simulink model "softMBD"  (R2025b)
settings: Solver=FixedStepAuto  StartTime=0.0  StopTime=30  FixedStep=0.005  RelTol=1e-3
values from neighbouring files (symbols this model uses):
  FPV_mass = 0.8    [Soft.m]
  g = 9.81    [Soft.m]
  ks = 0    [Soft.m]
  p_0 = 1013.25    [Soft.m]
  Q2Ts = forcetomotors()    [Soft.m]    (also in forcetomotors.m = inv(Ts2Q))
  takeOffDuration = 2    [Soft.m]
  Ts = 0.005    [Soft.m]
undefined symbols (not defined in the file or in its folder): CdA, DiscIntNeverNeededParam, kd_pq, kd_pr, kd_y, ki_pq, ki_pr, ki_y, kp_pq, kp_pr, kp_y, pInitialization, rho
libraries: simulink x37, discretizing x11, slpidlib x2, SignalEditorBlockLib x1, simulink_extras x1, shared6dof x1, dynamicsLibrary x1, aerolibasang x1, aerolibnav x1
(part 10 of 20)

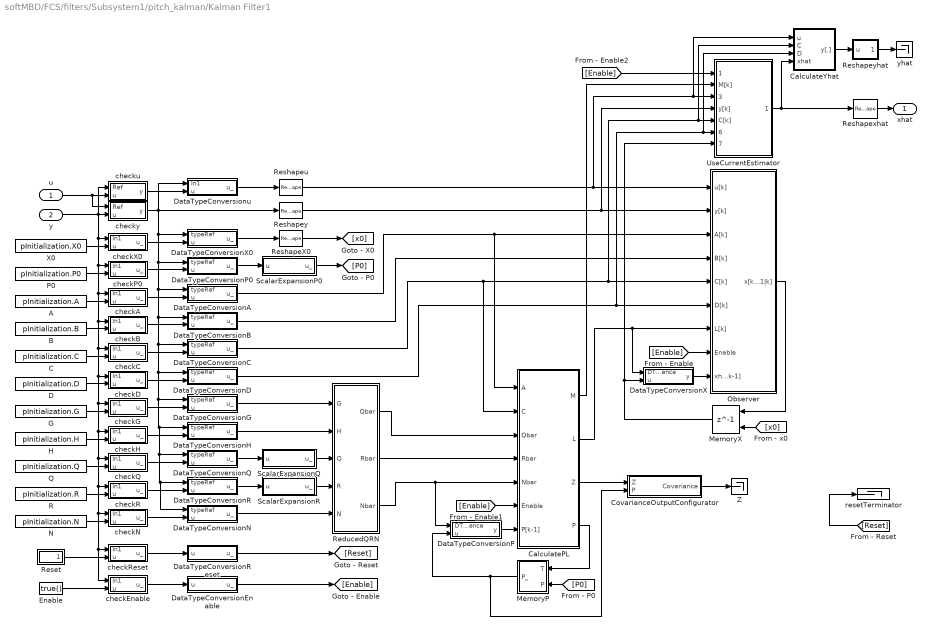
== system softMBD/FCS/filters/Subsystem1/pitch_kalman/Kalman Filter1 ==
  u : Inport
  y : Inport  Port=2
  A : Constant  Value=pInitialization.A  VectorParams1D=off  OutDataTypeStr=Inherit: Inherit via back propagation
  B : Constant  Value=pInitialization.B  VectorParams1D=off  OutDataTypeStr=Inherit: Inherit via back propagation
  C : Constant  Value=pInitialization.C  VectorParams1D=off  OutDataTypeStr=Inherit: Inherit via back propagation
  CalculatePL : Subsystem  AncestorBlock=ctrlSharedLib/KalmanFilterUtilities/ConstantPL  mask(ctrlKalmanFilterConstantPL){}
  CalculateYhat : Subsystem  AncestorBlock=ctrlSharedLib/KalmanFilterUtilities/DontCalculateYhat  mask(ctrlKalmanFilterDontCalculateYhat){}
  CovarianceOutputConfigurator : Subsystem
  D : Constant  Value=pInitialization.D  VectorParams1D=off  OutDataTypeStr=Inherit: Inherit via back propagation
  DataTypeConversionA : Subsystem  AncestorBlock=ctrlSharedLib/Utilities/DataTypeDuplicateAndOutput  mask(ctrlDataTypeDuplicateAndOutput){}
  DataTypeConversionB : Subsystem  AncestorBlock=ctrlSharedLib/Utilities/DataTypeDuplicateAndOutput  mask(ctrlDataTypeDuplicateAndOutput){}
  DataTypeConversionC : Subsystem  AncestorBlock=ctrlSharedLib/Utilities/DataTypeDuplicateAndOutput  mask(ctrlDataTypeDuplicateAndOutput){}
  DataTypeConversionD : Subsystem  AncestorBlock=ctrlSharedLib/Utilities/DataTypeDuplicateAndOutput  mask(ctrlDataTypeDuplicateAndOutput){}
  DataTypeConversionEnable : Subsystem  AncestorBlock=ctrlSharedLib/Utilities/PassInputThrough
  DataTypeConversionG : Subsystem  AncestorBlock=ctrlSharedLib/Utilities/DataTypeDuplicateAndOutput  mask(ctrlDataTypeDuplicateAndOutput){}
  DataTypeConversionH : Subsystem  AncestorBlock=ctrlSharedLib/Utilities/DataTypeDuplicateAndOutput  mask(ctrlDataTypeDuplicateAndOutput){}
  DataTypeConversionN : Subsystem  AncestorBlock=ctrlSharedLib/Utilities/DataTypeDuplicateAndOutput  mask(ctrlDataTypeDuplicateAndOutput){}
  DataTypeConversionP : Subsystem  AncestorBlock=|  mask(Conversion Inherited){ConvertRealWorld=Real World Value, RndMeth=Floor, DoSatur=off}
      | simulink/Signal
      | Attributes/Data Type
      | Conversion
      | Inherited
      mask prompts: ConvertRealWorld "Simulink:masks:InputAndOutputToHaveEqual_MP"; RndMeth "Simulink:masks:IntegerRoundingMode_MP"; DoSatur "Simulink:masks:SaturateToMaxOrMinWhenOverflowsOccur_MP"
      mask help: Simulink:masks:ConversionInherited_MD
      mask init:
      | rndMethCell = {'Ceiling','Convergent','Floor','Nearest','Round','Simplest','Zero'};
      | onOffCell = {'off','on'};
      | RWVvsSICell = { 'Real World Value','Stored Integer'};
      | set_param([gcb,'/Conversion'],'RndMeth',rndMethCell{RndMeth},...
      |                                 'DoSatur',onOffCell{DoSatur+1},...
      |                                 'ConvertRealWorld',RWVvsSICell{ConvertRealWorld});
      mask TypeOptions ConvertRealWorld: Simulink:masks:RealWorldValue | Simulink:masks:StoredInteger
      mask TypeOptions RndMeth: Simulink:masks:Ceiling | Simulink:masks:Convergent | Simulink:masks:Floor | Simulink:masks:Nearest | Simulink:masks:Round | Simulink:masks:Simplest | Simulink:masks:Zero
      mask Display:
      | port_label('Input',2,'u');
      | port_label('Output',1,'y');
      |     if(get_param(gcbh,'ConvertRealWorld') == "Stored Integer")
      |        disp('SI')
      |     else
      |        disp('Convert')
      |     end
  DataTypeConversionP0 : Subsystem  AncestorBlock=ctrlSharedLib/Utilities/DataTypeDuplicateAndOutput  mask(ctrlDataTypeDuplicateAndOutput){}
  DataTypeConversionQ : Subsystem  AncestorBlock=ctrlSharedLib/Utilities/DataTypeDuplicateAndOutput  mask(ctrlDataTypeDuplicateAndOutput){}
  DataTypeConversionR : Subsystem  AncestorBlock=ctrlSharedLib/Utilities/DataTypeDuplicateAndOutput  mask(ctrlDataTypeDuplicateAndOutput){}
  DataTypeConversionReset : Subsystem  AncestorBlock=ctrlSharedLib/Utilities/PassInputThrough
  DataTypeConversionX : Subsystem  AncestorBlock=|  mask(Conversion Inherited){ConvertRealWorld=Real World Value, RndMeth=Floor, DoSatur=off}
      | simulink/Signal
      | Attributes/Data Type
      | Conversion
      | Inherited
      mask prompts: ConvertRealWorld "Simulink:masks:InputAndOutputToHaveEqual_MP"; RndMeth "Simulink:masks:IntegerRoundingMode_MP"; DoSatur "Simulink:masks:SaturateToMaxOrMinWhenOverflowsOccur_MP"
      mask help: Simulink:masks:ConversionInherited_MD
      mask init: same as softMBD/FCS/filters/Subsystem1/pitch_kalman/Kalman Filter1/DataTypeConversionP
      mask TypeOptions ConvertRealWorld: Simulink:masks:RealWorldValue | Simulink:masks:StoredInteger
      mask TypeOptions RndMeth: Simulink:masks:Ceiling | Simulink:masks:Convergent | Simulink:masks:Floor | Simulink:masks:Nearest | Simulink:masks:Round | Simulink:masks:Simplest | Simulink:masks:Zero
      mask Display:
      | port_label('Input',2,'u');
      | port_label('Output',1,'y');
      |     if(get_param(gcbh,'ConvertRealWorld') == "Stored Integer")
      |        disp('SI')
      |     else
      |        disp('Convert')
      |     end
  DataTypeConversionX0 : Subsystem  AncestorBlock=ctrlSharedLib/Utilities/DataTypeDuplicateAndOutput  mask(ctrlDataTypeDuplicateAndOutput){}
  DataTypeConversionu : Subsystem  AncestorBlock=ctrlSharedLib/KalmanFilterUtilities/PassSecondInputThrough  mask(ctrlKalmanFilterPassSecondInputThrough){}
      mask Display:
      | port_label('Input',2,'u');
      | port_label('Output',1,'y');
  Enable : Constant  Value=true()  OutDataTypeStr=boolean
  G : Constant  Value=pInitialization.G  VectorParams1D=off  OutDataTypeStr=Inherit: Inherit via back propagation
  H : Constant  Value=pInitialization.H  VectorParams1D=off  OutDataTypeStr=Inherit: Inherit via back propagation
  MemoryP : Subsystem  AncestorBlock=ctrlSharedLib/KalmanFilterUtilities/MemoryP  mask(ctrlKalmanFilterNoMemoryP){}
      mask Display:
      | port_label('Input',2,'P');
      | port_label('Output',1,'P');
  MemoryX : Delay  DelayLength=1  InitialConditionSource=Input port  SampleTime=pInitialization.Ts
      settings: InputPortMap=u0,p4
  N : Constant  Value=pInitialization.N  VectorParams1D=off  OutDataTypeStr=Inherit: Inherit via back propagation
  Observer : Subsystem
  P0 : Constant  Value=pInitialization.P0  OutDataTypeStr=Inherit: Inherit via back propagation
  Q : Constant  Value=pInitialization.Q  VectorParams1D=off  OutDataTypeStr=Inherit: Inherit via back propagation
  R : Constant  Value=pInitialization.R  VectorParams1D=off  OutDataTypeStr=Inherit: Inherit via back propagation
  ReducedQRN : Subsystem  AncestorBlock=ctrlSharedLib/KalmanFilterUtilities/NoReducedQRN  mask(ctrlKalmanFilterNoReducedQRN){}
  Reset : Subsystem  AncestorBlock=ctrlSharedLib/Utilities/Ground  mask(ctrlSharedLibGround){OutDataTypeStr=boolean, Dimensions=1}
      mask prompts: OutDataTypeStr "Simulink:blkprm_prompts:UNIFIEDDATATYPE"; Dimensions "Simulink:blkprm_prompts:SigSpecDims"
      mask TypeOptions OutDataTypeStr: Signal Specification/OutDataTypeStr
      mask TypeOptions Dimensions: Signal Specification/Dimensions
      mask DialogControl OutDataTypeStr Prompt: Data type:
      mask DialogControl Dimensions Prompt: Dimensions (-1 for inherited):
  ReshapeX0 : Reshape
  Reshapeu : Reshape
  Reshapexhat : Reshape
  Reshapey : Reshape
  Reshapeyhat : Subsystem  AncestorBlock=ctrlSharedLib/Utilities/PassInputThrough
  ScalarExpansionP0 : Subsystem  AncestorBlock=ctrlSharedLib/Utilities/PassInputThrough
  ScalarExpansionQ : Subsystem  AncestorBlock=ctrlSharedLib/Utilities/PassInputThrough
  ScalarExpansionR : Subsystem  AncestorBlock=ctrlSharedLib/Utilities/PassInputThrough
  UseCurrentEstimator : Subsystem  AncestorBlock=ctrlSharedLib/KalmanFilterUtilities/UseCurrentEstimatorZeroD  mask(ctrlKalmanFilterUseCurrentEstimatorZeroD){}
  X0 : Constant  Value=pInitialization.X0  VectorParams1D=off  OutDataTypeStr=Inherit: Inherit via back propagation
  Z : Terminator
  checkA : Subsystem  AncestorBlock=ctrlSharedLib/KalmanFilterUtilities/PassSecondInputThrough  mask(ctrlKalmanFilterPassSecondInputThrough){}
      mask Display:
      | port_label('Input',2,'u');
      | port_label('Output',1,'y');
  checkB : Subsystem  AncestorBlock=ctrlSharedLib/KalmanFilterUtilities/PassSecondInputThrough  mask(ctrlKalmanFilterPassSecondInputThrough){}
      mask Display:
      | port_label('Input',2,'u');
      | port_label('Output',1,'y');
  checkC : Subsystem  AncestorBlock=ctrlSharedLib/KalmanFilterUtilities/PassSecondInputThrough  mask(ctrlKalmanFilterPassSecondInputThrough){}
      mask Display:
      | port_label('Input',2,'u');
      | port_label('Output',1,'y');
  checkD : Subsystem  AncestorBlock=ctrlSharedLib/KalmanFilterUtilities/PassSecondInputThrough  mask(ctrlKalmanFilterPassSecondInputThrough){}
      mask Display:
      | port_label('Input',2,'u');
      | port_label('Output',1,'y');
  checkEnable : Subsystem  AncestorBlock=ctrlSharedLib/KalmanFilterUtilities/PassSecondInputThrough  mask(ctrlKalmanFilterPassSecondInputThrough){}
      mask Display:
      | port_label('Input',2,'u');
      | port_label('Output',1,'y');
  checkG : Subsystem  AncestorBlock=ctrlSharedLib/KalmanFilterUtilities/PassSecondInputThrough  mask(ctrlKalmanFilterPassSecondInputThrough){}
      mask Display:
      | port_label('Input',2,'u');
      | port_label('Output',1,'y');
  checkH : Subsystem  AncestorBlock=ctrlSharedLib/KalmanFilterUtilities/PassSecondInputThrough  mask(ctrlKalmanFilterPassSecondInputThrough){}
      mask Display:
      | port_label('Input',2,'u');
      | port_label('Output',1,'y');
  checkN : Subsystem  AncestorBlock=ctrlSharedLib/KalmanFilterUtilities/PassSecondInputThrough  mask(ctrlKalmanFilterPassSecondInputThrough){}
      mask Display:
      | port_label('Input',2,'u');
      | port_label('Output',1,'y');
  checkP0 : Subsystem  AncestorBlock=ctrlSharedLib/KalmanFilterUtilities/PassSecondInputThrough  mask(ctrlKalmanFilterPassSecondInputThrough){}
      mask Display:
      | port_label('Input',2,'u');
      | port_label('Output',1,'y');
  checkQ : Subsystem  AncestorBlock=ctrlSharedLib/KalmanFilterUtilities/PassSecondInputThrough  mask(ctrlKalmanFilterPassSecondInputThrough){}
      mask Display:
      | port_label('Input',2,'u');
      | port_label('Output',1,'y');
  checkR : Subsystem  AncestorBlock=ctrlSharedLib/KalmanFilterUtilities/PassSecondInputThrough  mask(ctrlKalmanFilterPassSecondInputThrough){}
      mask Display:
      | port_label('Input',2,'u');
      | port_label('Output',1,'y');
  checkReset : Subsystem  AncestorBlock=ctrlSharedLib/KalmanFilterUtilities/PassSecondInputThrough  mask(ctrlKalmanFilterPassSecondInputThrough){}
      mask Display:
      | port_label('Input',2,'u');
      | port_label('Output',1,'y');
  checkX0 : Subsystem  AncestorBlock=ctrlSharedLib/KalmanFilterUtilities/PassSecondInputThrough  mask(ctrlKalmanFilterPassSecondInputThrough){}
      mask Display:
      | port_label('Input',2,'u');
      | port_label('Output',1,'y');
  checku : Subsystem  AncestorBlock=ctrlSharedLib/KalmanFilterUtilities/checkSignals  mask(ctrlKalmanFilterCheckSignals){Ts=pInitialization.Ts, Ns=pInitialization.Ns, Nu=pInitialization.Nu, Nw=pInitialization.Nw, Ny=pInitialization.Ny}
      mask prompts: Ts "Sample time:"; Ns "Number of states:"; Nu "Number of inputs:"; Nw "Number of process noise inputs:"; Ny "Number of outputs:"
      mask init:
      | Ns = int32(Ns);
      | Nu = int32(Nu);
      | Nw = int32(Nw);
      | Ny = int32(Ny);
      | 
      | lineH = get_param(gcbh,'LineHandles');
      | portName = get_param(get_param(lineH.Inport(2),'SrcBlockHandle'),'Name');
      | parentBlockPath = get_param(gcbh(),'Parent');
      | parentH = get_param(parentBlockPath,'Handle');
      | isContinuousTime = strcmp(get_param(parentH,'TimeDomain'),...
      |     slsvInternal('slsvGetEnStringFromCatalog','Controllib:blocks:maskPromptKFTimeDomainCT'));
      | clear lineH;
      mask DialogControl ParametersContainer Prompt: Parameters
  checky : Subsystem  AncestorBlock=ctrlSharedLib/KalmanFilterUtilities/checkSignals  mask(ctrlKalmanFilterCheckSignals){Ts=pInitialization.Ts, Ns=pInitialization.Ns, Nu=pInitialization.Nu, Nw=pInitialization.Nw, Ny=pInitialization.Ny}
      mask prompts: Ts "Sample time:"; Ns "Number of states:"; Nu "Number of inputs:"; Nw "Number of process noise inputs:"; Ny "Number of outputs:"
      mask init: same as softMBD/FCS/filters/Subsystem1/pitch_kalman/Kalman Filter1/checku
      mask DialogControl ParametersContainer Prompt: Parameters
  resetTerminator : Terminator
  yhat : Terminator
  xhat : Outport  VectorParamsAs1DForOutWhenUnconnected=off
  wires:
  [Reset] -> resetTerminator/1
  CalculatePL/3(Z) -> CovarianceOutputConfigurator/1(Z)
  Reshapexhat/1 -> xhat/1
  Reshapeyhat/1(u_) -> yhat/1
  UseCurrentEstimator/1(xhat[k|k]) -> Reshapexhat/1, CalculateYhat/4(xhat)
  checku/1(y) -> DataTypeConversionu/2(u)
  DataTypeConversionu/1(u_) -> Reshapeu/1
  CovarianceOutputConfigurator/1(Covariance) -> Z/1
  DataTypeConversionC/1(u_) -> Observer/5(C[k]), UseCurrentEstimator/5(C[k]), CalculateYhat/2(C), CalculatePL/2(C)
  ScalarExpansionR/1(u_) -> ReducedQRN/4(R)
  ScalarExpansionQ/1(u_) -> ReducedQRN/3(Q)
  ScalarExpansionP0/1(u_) -> [P0]
  CalculatePL/4(P) -> MemoryP/1(T)
  DataTypeConversionReset/1(u_) -> [Reset]
  checkReset/1(u_) -> DataTypeConversionReset/1(u)
  checky/1(y) -> DataTypeConversionX0/1(typeRef), DataTypeConversionP0/1(typeRef), DataTypeConversionC/1(typeRef), DataTypeConversionD/1(typeRef), DataTypeConversionG/1(typeRef), DataTypeConversionH/1(typeRef), DataTypeConversionQ/1(typeRef), DataTypeConversionR/1(typeRef), DataTypeConversionN/1(typeRef), DataTypeConversionB/1(typeRef), DataTypeConversionA/1(typeRef), Reshapey/1, DataTypeConversionu/1(In1)
  ReshapeX0/1 -> [x0]
  MemoryP/1(P_) -> DataTypeConversionP/2(u), CovarianceOutputConfigurator/2(P)
  [P0] -> MemoryP/2(P)
  CalculateYhat/1(y[.]) -> Reshapeyhat/1(u)
  [Enable] -> UseCurrentEstimator/1(Enable[k])
  CalculatePL/1(M) -> UseCurrentEstimator/2(M[k])
  CalculatePL/2(L) -> Observer/7(L[k]), DataTypeConversionX/1(DTS reference)
  Reshapey/1 -> Observer/2(y[k]), UseCurrentEstimator/4(y[k])
  Reshapeu/1 -> Observer/1(u[k]), UseCurrentEstimator/3(u (unused)), CalculateYhat/1(u)
  y/1 -> checky/2(u), checku/1(Ref), checkX0/1(In1), checkP0/1(In1), checkA/1(In1), checkB/1(In1), checkC/1(In1), checkD/1(In1), checkG/1(In1), checkH/1(In1), checkQ/1(In1), checkR/1(In1), checkN/1(In1), checkReset/1(In1), checkEnable/1(In1)
  u/1 -> checku/2(u), checky/1(Ref)
  DataTypeConversionP/1(y) -> CalculatePL/7(P[k-1])
  [Enable] -> Observer/8(Enable)
  DataTypeConversionX/1(y) -> Observer/9(xhat[k|k-1])
  DataTypeConversionX0/1(u_) -> ReshapeX0/1
  [x0] -> MemoryX/2
  X0/1 -> checkX0/2(u)
  DataTypeConversionD/1(u_) -> Observer/6(D[k]), UseCurrentEstimator/6(D (unused)), CalculateYhat/3(D)
  DataTypeConversionB/1(u_) -> Observer/4(B[k])
  DataTypeConversionA/1(u_) -> Observer/3(A[k]), CalculatePL/1(A)
  checkB/1(u_) -> DataTypeConversionB/2(u)
  B/1 -> checkB/2(u)
  ReducedQRN/3(Nbar) -> CalculatePL/5(Nbar), DataTypeConversionP/1(DTS reference)
  ReducedQRN/2(Rbar) -> CalculatePL/4(Rbar)
  ReducedQRN/1(Qbar) -> CalculatePL/3(Qbar)
  checkA/1(u_) -> DataTypeConversionA/2(u)
  A/1 -> checkA/2(u)
  [Enable] -> CalculatePL/6(Enable)
  Observer/1(x[k+1|k]) -> MemoryX/1
  DataTypeConversionEnable/1(u_) -> [Enable]
  checkEnable/1(u_) -> DataTypeConversionEnable/1(u)
  Enable/1 -> checkEnable/2(u)
  DataTypeConversionP0/1(u_) -> ScalarExpansionP0/1(u)
  Reset/1(Out) -> checkReset/2(u)
  DataTypeConversionN/1(u_) -> ReducedQRN/5(N)
  checkN/1(u_) -> DataTypeConversionN/2(u)
  checkR/1(u_) -> DataTypeConversionR/2(u)
  DataTypeConversionR/1(u_) -> ScalarExpansionR/1(u)
  checkQ/1(u_) -> DataTypeConversionQ/2(u)
  DataTypeConversionQ/1(u_) -> ScalarExpansionQ/1(u)
  DataTypeConversionH/1(u_) -> ReducedQRN/2(H)
  checkH/1(u_) -> DataTypeConversionH/2(u)
  DataTypeConversionG/1(u_) -> ReducedQRN/1(G)
  checkG/1(u_) -> DataTypeConversionG/2(u)
  checkD/1(u_) -> DataTypeConversionD/2(u)
  checkC/1(u_) -> DataTypeConversionC/2(u)
  checkP0/1(u_) -> DataTypeConversionP0/2(u)
  checkX0/1(u_) -> DataTypeConversionX0/2(u)
  MemoryX/1 -> DataTypeConversionX/2(u), UseCurrentEstimator/7(xhat[k|k-1])
  N/1 -> checkN/2(u)
  R/1 -> checkR/2(u)
  Q/1 -> checkQ/2(u)
  H/1 -> checkH/2(u)
  G/1 -> checkG/2(u)
  D/1 -> checkD/2(u)
  P0/1 -> checkP0/2(u)
  C/1 -> checkC/2(u)

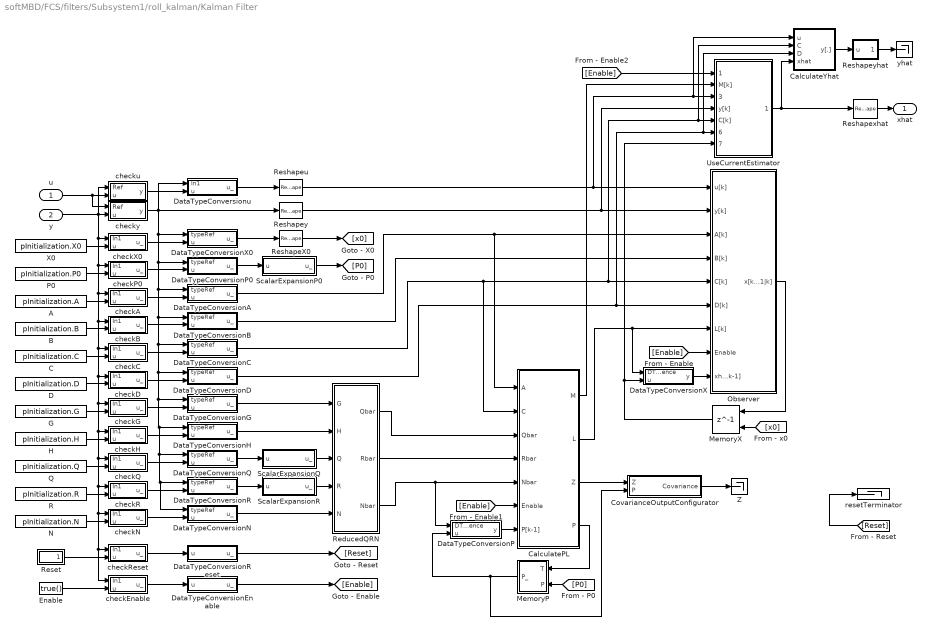
== system softMBD/FCS/filters/Subsystem1/roll_kalman/Kalman Filter ==
  u : Inport
  y : Inport  Port=2
  A : Constant  Value=pInitialization.A  VectorParams1D=off  OutDataTypeStr=Inherit: Inherit via back propagation
  B : Constant  Value=pInitialization.B  VectorParams1D=off  OutDataTypeStr=Inherit: Inherit via back propagation
  C : Constant  Value=pInitialization.C  VectorParams1D=off  OutDataTypeStr=Inherit: Inherit via back propagation
  CalculatePL : Subsystem  AncestorBlock=ctrlSharedLib/KalmanFilterUtilities/ConstantPL  mask(ctrlKalmanFilterConstantPL){}
  CalculateYhat : Subsystem  AncestorBlock=ctrlSharedLib/KalmanFilterUtilities/DontCalculateYhat  mask(ctrlKalmanFilterDontCalculateYhat){}
  CovarianceOutputConfigurator : Subsystem
  D : Constant  Value=pInitialization.D  VectorParams1D=off  OutDataTypeStr=Inherit: Inherit via back propagation
  DataTypeConversionA : Subsystem  AncestorBlock=ctrlSharedLib/Utilities/DataTypeDuplicateAndOutput  mask(ctrlDataTypeDuplicateAndOutput){}
  DataTypeConversionB : Subsystem  AncestorBlock=ctrlSharedLib/Utilities/DataTypeDuplicateAndOutput  mask(ctrlDataTypeDuplicateAndOutput){}
  DataTypeConversionC : Subsystem  AncestorBlock=ctrlSharedLib/Utilities/DataTypeDuplicateAndOutput  mask(ctrlDataTypeDuplicateAndOutput){}
  DataTypeConversionD : Subsystem  AncestorBlock=ctrlSharedLib/Utilities/DataTypeDuplicateAndOutput  mask(ctrlDataTypeDuplicateAndOutput){}
  DataTypeConversionEnable : Subsystem  AncestorBlock=ctrlSharedLib/Utilities/PassInputThrough
  DataTypeConversionG : Subsystem  AncestorBlock=ctrlSharedLib/Utilities/DataTypeDuplicateAndOutput  mask(ctrlDataTypeDuplicateAndOutput){}
  DataTypeConversionH : Subsystem  AncestorBlock=ctrlSharedLib/Utilities/DataTypeDuplicateAndOutput  mask(ctrlDataTypeDuplicateAndOutput){}
  DataTypeConversionN : Subsystem  AncestorBlock=ctrlSharedLib/Utilities/DataTypeDuplicateAndOutput  mask(ctrlDataTypeDuplicateAndOutput){}
  DataTypeConversionP : Subsystem  AncestorBlock=|  mask(Conversion Inherited){ConvertRealWorld=Real World Value, RndMeth=Floor, DoSatur=off}
      | simulink/Signal
      | Attributes/Data Type
      | Conversion
      | Inherited
      mask prompts: ConvertRealWorld "Simulink:masks:InputAndOutputToHaveEqual_MP"; RndMeth "Simulink:masks:IntegerRoundingMode_MP"; DoSatur "Simulink:masks:SaturateToMaxOrMinWhenOverflowsOccur_MP"
      mask help: Simulink:masks:ConversionInherited_MD
      mask init: same as softMBD/FCS/filters/Subsystem1/pitch_kalman/Kalman Filter1/DataTypeConversionP
      mask TypeOptions ConvertRealWorld: Simulink:masks:RealWorldValue | Simulink:masks:StoredInteger
      mask TypeOptions RndMeth: Simulink:masks:Ceiling | Simulink:masks:Convergent | Simulink:masks:Floor | Simulink:masks:Nearest | Simulink:masks:Round | Simulink:masks:Simplest | Simulink:masks:Zero
      mask Display:
      | port_label('Input',2,'u');
      | port_label('Output',1,'y');
      |     if(get_param(gcbh,'ConvertRealWorld') == "Stored Integer")
      |        disp('SI')
      |     else
      |        disp('Convert')
      |     end
  DataTypeConversionP0 : Subsystem  AncestorBlock=ctrlSharedLib/Utilities/DataTypeDuplicateAndOutput  mask(ctrlDataTypeDuplicateAndOutput){}
  DataTypeConversionQ : Subsystem  AncestorBlock=ctrlSharedLib/Utilities/DataTypeDuplicateAndOutput  mask(ctrlDataTypeDuplicateAndOutput){}
  DataTypeConversionR : Subsystem  AncestorBlock=ctrlSharedLib/Utilities/DataTypeDuplicateAndOutput  mask(ctrlDataTypeDuplicateAndOutput){}
  DataTypeConversionReset : Subsystem  AncestorBlock=ctrlSharedLib/Utilities/PassInputThrough
  DataTypeConversionX : Subsystem  AncestorBlock=|  mask(Conversion Inherited){ConvertRealWorld=Real World Value, RndMeth=Floor, DoSatur=off}
      | simulink/Signal
      | Attributes/Data Type
      | Conversion
      | Inherited
      mask prompts: ConvertRealWorld "Simulink:masks:InputAndOutputToHaveEqual_MP"; RndMeth "Simulink:masks:IntegerRoundingMode_MP"; DoSatur "Simulink:masks:SaturateToMaxOrMinWhenOverflowsOccur_MP"
      mask help: Simulink:masks:ConversionInherited_MD
      mask init: same as softMBD/FCS/filters/Subsystem1/pitch_kalman/Kalman Filter1/DataTypeConversionP
      mask TypeOptions ConvertRealWorld: Simulink:masks:RealWorldValue | Simulink:masks:StoredInteger
      mask TypeOptions RndMeth: Simulink:masks:Ceiling | Simulink:masks:Convergent | Simulink:masks:Floor | Simulink:masks:Nearest | Simulink:masks:Round | Simulink:masks:Simplest | Simulink:masks:Zero
      mask Display:
      | port_label('Input',2,'u');
      | port_label('Output',1,'y');
      |     if(get_param(gcbh,'ConvertRealWorld') == "Stored Integer")
      |        disp('SI')
      |     else
      |        disp('Convert')
      |     end
  DataTypeConversionX0 : Subsystem  AncestorBlock=ctrlSharedLib/Utilities/DataTypeDuplicateAndOutput  mask(ctrlDataTypeDuplicateAndOutput){}
  DataTypeConversionu : Subsystem  AncestorBlock=ctrlSharedLib/KalmanFilterUtilities/PassSecondInputThrough  mask(ctrlKalmanFilterPassSecondInputThrough){}
      mask Display:
      | port_label('Input',2,'u');
      | port_label('Output',1,'y');
  Enable : Constant  Value=true()  OutDataTypeStr=boolean
  G : Constant  Value=pInitialization.G  VectorParams1D=off  OutDataTypeStr=Inherit: Inherit via back propagation
  H : Constant  Value=pInitialization.H  VectorParams1D=off  OutDataTypeStr=Inherit: Inherit via back propagation
  MemoryP : Subsystem  AncestorBlock=ctrlSharedLib/KalmanFilterUtilities/MemoryP  mask(ctrlKalmanFilterNoMemoryP){}
      mask Display:
      | port_label('Input',2,'P');
      | port_label('Output',1,'P');
  MemoryX : Delay  DelayLength=1  InitialConditionSource=Input port  SampleTime=pInitialization.Ts
      settings: InputPortMap=u0,p4
  N : Constant  Value=pInitialization.N  VectorParams1D=off  OutDataTypeStr=Inherit: Inherit via back propagation
  Observer : Subsystem
  P0 : Constant  Value=pInitialization.P0  OutDataTypeStr=Inherit: Inherit via back propagation
  Q : Constant  Value=pInitialization.Q  VectorParams1D=off  OutDataTypeStr=Inherit: Inherit via back propagation
  R : Constant  Value=pInitialization.R  VectorParams1D=off  OutDataTypeStr=Inherit: Inherit via back propagation
  ReducedQRN : Subsystem  AncestorBlock=ctrlSharedLib/KalmanFilterUtilities/NoReducedQRN  mask(ctrlKalmanFilterNoReducedQRN){}
  Reset : Subsystem  AncestorBlock=ctrlSharedLib/Utilities/Ground  mask(ctrlSharedLibGround){OutDataTypeStr=boolean, Dimensions=1}
      mask prompts: OutDataTypeStr "Simulink:blkprm_prompts:UNIFIEDDATATYPE"; Dimensions "Simulink:blkprm_prompts:SigSpecDims"
      mask TypeOptions OutDataTypeStr: Signal Specification/OutDataTypeStr
      mask TypeOptions Dimensions: Signal Specification/Dimensions
      mask DialogControl OutDataTypeStr Prompt: Data type:
      mask DialogControl Dimensions Prompt: Dimensions (-1 for inherited):
  ReshapeX0 : Reshape
  Reshapeu : Reshape
  Reshapexhat : Reshape
  Reshapey : Reshape
  Reshapeyhat : Subsystem  AncestorBlock=ctrlSharedLib/Utilities/PassInputThrough
  ScalarExpansionP0 : Subsystem  AncestorBlock=ctrlSharedLib/Utilities/PassInputThrough
  ScalarExpansionQ : Subsystem  AncestorBlock=ctrlSharedLib/Utilities/PassInputThrough
  ScalarExpansionR : Subsystem  AncestorBlock=ctrlSharedLib/Utilities/PassInputThrough
  UseCurrentEstimator : Subsystem  AncestorBlock=ctrlSharedLib/KalmanFilterUtilities/UseCurrentEstimatorZeroD  mask(ctrlKalmanFilterUseCurrentEstimatorZeroD){}
  X0 : Constant  Value=pInitialization.X0  VectorParams1D=off  OutDataTypeStr=Inherit: Inherit via back propagation
  Z : Terminator
  checkA : Subsystem  AncestorBlock=ctrlSharedLib/KalmanFilterUtilities/PassSecondInputThrough  mask(ctrlKalmanFilterPassSecondInputThrough){}
      mask Display:
      | port_label('Input',2,'u');
      | port_label('Output',1,'y');
  checkB : Subsystem  AncestorBlock=ctrlSharedLib/KalmanFilterUtilities/PassSecondInputThrough  mask(ctrlKalmanFilterPassSecondInputThrough){}
      mask Display:
      | port_label('Input',2,'u');
      | port_label('Output',1,'y');
  checkC : Subsystem  AncestorBlock=ctrlSharedLib/KalmanFilterUtilities/PassSecondInputThrough  mask(ctrlKalmanFilterPassSecondInputThrough){}
      mask Display:
      | port_label('Input',2,'u');
      | port_label('Output',1,'y');
  checkD : Subsystem  AncestorBlock=ctrlSharedLib/KalmanFilterUtilities/PassSecondInputThrough  mask(ctrlKalmanFilterPassSecondInputThrough){}
      mask Display:
      | port_label('Input',2,'u');
      | port_label('Output',1,'y');
  checkEnable : Subsystem  AncestorBlock=ctrlSharedLib/KalmanFilterUtilities/PassSecondInputThrough  mask(ctrlKalmanFilterPassSecondInputThrough){}
      mask Display:
      | port_label('Input',2,'u');
      | port_label('Output',1,'y');
  checkG : Subsystem  AncestorBlock=ctrlSharedLib/KalmanFilterUtilities/PassSecondInputThrough  mask(ctrlKalmanFilterPassSecondInputThrough){}
      mask Display:
      | port_label('Input',2,'u');
      | port_label('Output',1,'y');
  checkH : Subsystem  AncestorBlock=ctrlSharedLib/KalmanFilterUtilities/PassSecondInputThrough  mask(ctrlKalmanFilterPassSecondInputThrough){}
      mask Display:
      | port_label('Input',2,'u');
      | port_label('Output',1,'y');
  checkN : Subsystem  AncestorBlock=ctrlSharedLib/KalmanFilterUtilities/PassSecondInputThrough  mask(ctrlKalmanFilterPassSecondInputThrough){}
      mask Display:
      | port_label('Input',2,'u');
      | port_label('Output',1,'y');
  checkP0 : Subsystem  AncestorBlock=ctrlSharedLib/KalmanFilterUtilities/PassSecondInputThrough  mask(ctrlKalmanFilterPassSecondInputThrough){}
      mask Display:
      | port_label('Input',2,'u');
      | port_label('Output',1,'y');
  checkQ : Subsystem  AncestorBlock=ctrlSharedLib/KalmanFilterUtilities/PassSecondInputThrough  mask(ctrlKalmanFilterPassSecondInputThrough){}
      mask Display:
      | port_label('Input',2,'u');
      | port_label('Output',1,'y');
  checkR : Subsystem  AncestorBlock=ctrlSharedLib/KalmanFilterUtilities/PassSecondInputThrough  mask(ctrlKalmanFilterPassSecondInputThrough){}
      mask Display:
      | port_label('Input',2,'u');
      | port_label('Output',1,'y');
  checkReset : Subsystem  AncestorBlock=ctrlSharedLib/KalmanFilterUtilities/PassSecondInputThrough  mask(ctrlKalmanFilterPassSecondInputThrough){}
      mask Display:
      | port_label('Input',2,'u');
      | port_label('Output',1,'y');
  checkX0 : Subsystem  AncestorBlock=ctrlSharedLib/KalmanFilterUtilities/PassSecondInputThrough  mask(ctrlKalmanFilterPassSecondInputThrough){}
      mask Display:
      | port_label('Input',2,'u');
      | port_label('Output',1,'y');
  checku : Subsystem  AncestorBlock=ctrlSharedLib/KalmanFilterUtilities/checkSignals  mask(ctrlKalmanFilterCheckSignals){Ts=pInitialization.Ts, Ns=pInitialization.Ns, Nu=pInitialization.Nu, Nw=pInitialization.Nw, Ny=pInitialization.Ny}
      mask prompts: Ts "Sample time:"; Ns "Number of states:"; Nu "Number of inputs:"; Nw "Number of process noise inputs:"; Ny "Number of outputs:"
      mask init: same as softMBD/FCS/filters/Subsystem1/pitch_kalman/Kalman Filter1/checku
      mask DialogControl ParametersContainer Prompt: Parameters
  checky : Subsystem  AncestorBlock=ctrlSharedLib/KalmanFilterUtilities/checkSignals  mask(ctrlKalmanFilterCheckSignals){Ts=pInitialization.Ts, Ns=pInitialization.Ns, Nu=pInitialization.Nu, Nw=pInitialization.Nw, Ny=pInitialization.Ny}
      mask prompts: Ts "Sample time:"; Ns "Number of states:"; Nu "Number of inputs:"; Nw "Number of process noise inputs:"; Ny "Number of outputs:"
      mask init: same as softMBD/FCS/filters/Subsystem1/pitch_kalman/Kalman Filter1/checku
      mask DialogControl ParametersContainer Prompt: Parameters
  resetTerminator : Terminator
  yhat : Terminator
  xhat : Outport  VectorParamsAs1DForOutWhenUnconnected=off
  wires:
  [Reset] -> resetTerminator/1
  CalculatePL/3(Z) -> CovarianceOutputConfigurator/1(Z)
  Reshapexhat/1 -> xhat/1
  Reshapeyhat/1(u_) -> yhat/1
  UseCurrentEstimator/1(xhat[k|k]) -> Reshapexhat/1, CalculateYhat/4(xhat)
  checku/1(y) -> DataTypeConversionu/2(u)
  DataTypeConversionu/1(u_) -> Reshapeu/1
  CovarianceOutputConfigurator/1(Covariance) -> Z/1
  DataTypeConversionC/1(u_) -> Observer/5(C[k]), UseCurrentEstimator/5(C[k]), CalculateYhat/2(C), CalculatePL/2(C)
  ScalarExpansionR/1(u_) -> ReducedQRN/4(R)
  ScalarExpansionQ/1(u_) -> ReducedQRN/3(Q)
  ScalarExpansionP0/1(u_) -> [P0]
  CalculatePL/4(P) -> MemoryP/1(T)
  DataTypeConversionReset/1(u_) -> [Reset]
  checkReset/1(u_) -> DataTypeConversionReset/1(u)
  checky/1(y) -> DataTypeConversionX0/1(typeRef), DataTypeConversionP0/1(typeRef), DataTypeConversionC/1(typeRef), DataTypeConversionD/1(typeRef), DataTypeConversionG/1(typeRef), DataTypeConversionH/1(typeRef), DataTypeConversionQ/1(typeRef), DataTypeConversionR/1(typeRef), DataTypeConversionN/1(typeRef), DataTypeConversionB/1(typeRef), DataTypeConversionA/1(typeRef), Reshapey/1, DataTypeConversionu/1(In1)
  ReshapeX0/1 -> [x0]
  MemoryP/1(P_) -> DataTypeConversionP/2(u), CovarianceOutputConfigurator/2(P)
  [P0] -> MemoryP/2(P)
  CalculateYhat/1(y[.]) -> Reshapeyhat/1(u)
  [Enable] -> UseCurrentEstimator/1(Enable[k])
  CalculatePL/1(M) -> UseCurrentEstimator/2(M[k])
  CalculatePL/2(L) -> Observer/7(L[k]), DataTypeConversionX/1(DTS reference)
  Reshapey/1 -> Observer/2(y[k]), UseCurrentEstimator/4(y[k])
  Reshapeu/1 -> Observer/1(u[k]), UseCurrentEstimator/3(u (unused)), CalculateYhat/1(u)
  y/1 -> checky/2(u), checku/1(Ref), checkX0/1(In1), checkP0/1(In1), checkA/1(In1), checkB/1(In1), checkC/1(In1), checkD/1(In1), checkG/1(In1), checkH/1(In1), checkQ/1(In1), checkR/1(In1), checkN/1(In1), checkReset/1(In1), checkEnable/1(In1)
  u/1 -> checku/2(u), checky/1(Ref)
  DataTypeConversionP/1(y) -> CalculatePL/7(P[k-1])
  [Enable] -> Observer/8(Enable)
  DataTypeConversionX/1(y) -> Observer/9(xhat[k|k-1])
  DataTypeConversionX0/1(u_) -> ReshapeX0/1
  [x0] -> MemoryX/2
  X0/1 -> checkX0/2(u)
  DataTypeConversionD/1(u_) -> Observer/6(D[k]), UseCurrentEstimator/6(D (unused)), CalculateYhat/3(D)
  DataTypeConversionB/1(u_) -> Observer/4(B[k])
  DataTypeConversionA/1(u_) -> Observer/3(A[k]), CalculatePL/1(A)
  checkB/1(u_) -> DataTypeConversionB/2(u)
  B/1 -> checkB/2(u)
  ReducedQRN/3(Nbar) -> CalculatePL/5(Nbar), DataTypeConversionP/1(DTS reference)
  ReducedQRN/2(Rbar) -> CalculatePL/4(Rbar)
  ReducedQRN/1(Qbar) -> CalculatePL/3(Qbar)
  checkA/1(u_) -> DataTypeConversionA/2(u)
  A/1 -> checkA/2(u)
  [Enable] -> CalculatePL/6(Enable)
  Observer/1(x[k+1|k]) -> MemoryX/1
  DataTypeConversionEnable/1(u_) -> [Enable]
  checkEnable/1(u_) -> DataTypeConversionEnable/1(u)
  Enable/1 -> checkEnable/2(u)
  DataTypeConversionP0/1(u_) -> ScalarExpansionP0/1(u)
  Reset/1(Out) -> checkReset/2(u)
  DataTypeConversionN/1(u_) -> ReducedQRN/5(N)
  checkN/1(u_) -> DataTypeConversionN/2(u)
  checkR/1(u_) -> DataTypeConversionR/2(u)
  DataTypeConversionR/1(u_) -> ScalarExpansionR/1(u)
  checkQ/1(u_) -> DataTypeConversionQ/2(u)
  DataTypeConversionQ/1(u_) -> ScalarExpansionQ/1(u)
  DataTypeConversionH/1(u_) -> ReducedQRN/2(H)
  checkH/1(u_) -> DataTypeConversionH/2(u)
  DataTypeConversionG/1(u_) -> ReducedQRN/1(G)
  checkG/1(u_) -> DataTypeConversionG/2(u)
  checkD/1(u_) -> DataTypeConversionD/2(u)
  checkC/1(u_) -> DataTypeConversionC/2(u)
  checkP0/1(u_) -> DataTypeConversionP0/2(u)
  checkX0/1(u_) -> DataTypeConversionX0/2(u)
  MemoryX/1 -> DataTypeConversionX/2(u), UseCurrentEstimator/7(xhat[k|k-1])
  N/1 -> checkN/2(u)
  R/1 -> checkR/2(u)
  Q/1 -> checkQ/2(u)
  H/1 -> checkH/2(u)
  G/1 -> checkG/2(u)
  D/1 -> checkD/2(u)
  P0/1 -> checkP0/2(u)
  C/1 -> checkC/2(u)

== system softMBD/FCS/Controller/position_controller/PID Controller/Anti-windup/Back Calculation ==
  preSat : Inport  SampleTime=SampleTime
  postSat : Inport  Port=2  SampleTime=SampleTime
  preInt : Inport  Port=3  SampleTime=SampleTime
  P : Inport  Port=4  SampleTime=SampleTime
  Kb : Gain  Gain=Kb  ParamMin=KbParamMin  ParamMax=KbParamMax  OutMin=KbOutMin  OutMax=KbOutMax
  Signal Specification2 : SignalSpecification  DisableCoverage=on  OutDataTypeStr=boolean  SampleTime=SampleTime
  SumI2 : Sum  DisableCoverage=on  Inputs=|-+  OutMin=SumI2OutMin  OutMax=SumI2OutMax
  SumI4 : Sum  DisableCoverage=on  Inputs=|++  OutMin=SumI4OutMin  OutMax=SumI4OutMax
  Terminator2 : Terminator
  Out1 : Outport  SampleTime=SampleTime
  wires:
  preSat/1 -> SumI2/1
  postSat/1 -> SumI2/2
  SumI2/1 -> Kb/1
  Kb/1 -> SumI4/1
  SumI4/1 -> Out1/1
  preInt/1 -> SumI4/2
  Signal Specification2/1 -> Terminator2/1
  P/1 -> Signal Specification2/1

== system softMBD/FCS/Controller/position_controller/PID Controller/Anti-windup/Cont. Clamping Ideal ==
  preSat : Inport  SampleTime=SampleTime
  P : Inport  Port=2  SampleTime=SampleTime
  preInt : Inport  Port=3  SampleTime=SampleTime
  postSat : Inport  Port=4  SampleTime=SampleTime
  Upper Limit : Inport  Port=5  SampleTime=SampleTime
  Lower Limit : Inport  Port=6  SampleTime=SampleTime
  AND1 : Logic  DisableCoverage=on  OutDataTypeStr=boolean
  AND2 : Logic  DisableCoverage=on  OutDataTypeStr=boolean
  AND3 : Logic  DisableCoverage=on  OutDataTypeStr=boolean
  Constant : Constant  DisableCoverage=on  OutDataTypeStr=int8  PreserveConstantTs=on
  Constant1 : Constant  DisableCoverage=on  Value=0  OutDataTypeStr=Inherit: Inherit via back propagation  PreserveConstantTs=on
  DataTypeConv1 : DataTypeConversion  DisableCoverage=on  OutDataTypeStr=int8  SaturateOnIntegerOverflow=off  RndMeth=Floor
  DataTypeConv2 : DataTypeConversion  DisableCoverage=on  OutDataTypeStr=int8  SaturateOnIntegerOverflow=off  RndMeth=Floor
  DataTypeConv4 : DataTypeConversion  DisableCoverage=on  OutDataTypeStr=int8  SaturateOnIntegerOverflow=off  RndMeth=Floor
  Dead Zone : Subsystem  Variant=on  VariantControlMode=label  LabelModeActiveChoice=Enabled  EmptyChoice=on
  Equal1 : RelationalOperator  DisableCoverage=on  Operator===  OutDataTypeStr=boolean  RndMeth=Floor  InputSameDT=off
  Equal2 : RelationalOperator  DisableCoverage=on  Operator===  OutDataTypeStr=boolean  RndMeth=Floor  InputSameDT=off
  Memory : Memory  DisableCoverage=on  InheritSampleTime=on
  NOT1 : Logic  DisableCoverage=on  Operator=NOT  OutDataTypeStr=boolean
  NOT2 : Logic  DisableCoverage=on  Operator=NOT  OutDataTypeStr=boolean
  NotEqual : RelationalOperator  DisableCoverage=on  Operator=~=  OutDataTypeStr=boolean  RndMeth=Floor  InputSameDT=off
  OR1 : Logic  DisableCoverage=on  Operator=OR  OutDataTypeStr=boolean
  SignP : Signum  DisableCoverage=on
  SignPreIntegrator : Signum  DisableCoverage=on
  SignPreSat : Signum  DisableCoverage=on
  Switch : Switch  Criteria=u2 > Threshold  SaturateOnIntegerOverflow=off
  Terminator1 : Terminator
  ZeroGain : Gain  DisableCoverage=on  Gain=0  OutDataTypeStr=Inherit: Same as input  ParamDataTypeStr=Inherit: Same as input
  Out1 : Outport  SampleTime=SampleTime
  wires:
  Upper Limit/1 -> Dead Zone/2(Upper Limit)
  Lower Limit/1 -> Dead Zone/3(Lower Limit)
  DataTypeConv4/1 -> Equal2/2
  Constant/1 -> Equal2/1
  DataTypeConv2/1 -> Equal1/2
  DataTypeConv1/1 -> Equal1/1
  AND3/1 -> Memory/1
  OR1/1 -> AND3/2
  AND2/1 -> OR1/2
  AND1/1 -> OR1/1
  NOT2/1 -> AND2/2
  NOT1/1 -> AND2/1
  Equal2/1 -> NOT2/1, AND1/2
  Equal1/1 -> AND1/1, NOT1/1
  NotEqual/1 -> AND3/1
  SignP/1 -> DataTypeConv4/1
  SignPreIntegrator/1 -> DataTypeConv2/1
  SignPreSat/1 -> DataTypeConv1/1
  P/1 -> SignP/1
  preInt/1 -> Switch/3, SignPreIntegrator/1
  Dead Zone/1(DZ out) -> SignPreSat/1, NotEqual/2
  ZeroGain/1 -> NotEqual/1
  preSat/1 -> ZeroGain/1, Dead Zone/1(preSat)
  Switch/1 -> Out1/1
  Constant1/1 -> Switch/1
  Memory/1 -> Switch/2
  postSat/1 -> Terminator1/1

== system softMBD/FCS/Controller/position_controller/PID Controller/Anti-windup/Cont. Clamping Parallel ==
  preSat : Inport  SampleTime=SampleTime
  preInt : Inport  Port=2  SampleTime=SampleTime
  postSat : Inport  Port=3  SampleTime=SampleTime
  P : Inport  Port=4  SampleTime=SampleTime
  Upper Limit : Inport  Port=5  SampleTime=SampleTime
  Lower Limit : Inport  Port=6  SampleTime=SampleTime
  AND3 : Logic  DisableCoverage=on  OutDataTypeStr=boolean
  Constant1 : Constant  DisableCoverage=on  Value=0  OutDataTypeStr=Inherit: Inherit via back propagation  PreserveConstantTs=on
  DataTypeConv1 : DataTypeConversion  DisableCoverage=on  OutDataTypeStr=int8  SaturateOnIntegerOverflow=off  RndMeth=Floor
  DataTypeConv2 : DataTypeConversion  DisableCoverage=on  OutDataTypeStr=int8  SaturateOnIntegerOverflow=off  RndMeth=Floor
  Dead Zone : Subsystem  Variant=on  VariantControlMode=label  LabelModeActiveChoice=Enabled  EmptyChoice=on
  Equal1 : RelationalOperator  DisableCoverage=on  Operator===  OutDataTypeStr=boolean  RndMeth=Floor  InputSameDT=off
  Memory : Memory  DisableCoverage=on  InheritSampleTime=on
  NotEqual : RelationalOperator  DisableCoverage=on  Operator=~=  OutDataTypeStr=boolean  RndMeth=Floor  InputSameDT=off
  SignPreIntegrator : Signum  DisableCoverage=on
  SignPreSat : Signum  DisableCoverage=on
  Signal Specification2 : SignalSpecification  DisableCoverage=on  OutDataTypeStr=boolean  SampleTime=SampleTime
  Switch : Switch  Criteria=u2 > Threshold  SaturateOnIntegerOverflow=off
  Terminator1 : Terminator
  Terminator2 : Terminator
  ZeroGain : Gain  DisableCoverage=on  Gain=0  OutDataTypeStr=Inherit: Same as input  ParamDataTypeStr=Inherit: Same as input
  Out1 : Outport  SampleTime=SampleTime
  wires:
  Upper Limit/1 -> Dead Zone/2(Upper Limit)
  Lower Limit/1 -> Dead Zone/3(Lower Limit)
  AND3/1 -> Memory/1
  Constant1/1 -> Switch/1
  DataTypeConv2/1 -> Equal1/2
  DataTypeConv1/1 -> Equal1/1
  Equal1/1 -> AND3/2
  NotEqual/1 -> AND3/1
  SignPreIntegrator/1 -> DataTypeConv2/1
  SignPreSat/1 -> DataTypeConv1/1
  preInt/1 -> SignPreIntegrator/1, Switch/3
  Dead Zone/1(DZ out) -> SignPreSat/1, NotEqual/2
  ZeroGain/1 -> NotEqual/1
  preSat/1 -> ZeroGain/1, Dead Zone/1(preSat)
  Switch/1 -> Out1/1
  Memory/1 -> Switch/2
  Signal Specification2/1 -> Terminator2/1
  postSat/1 -> Terminator1/1
  P/1 -> Signal Specification2/1

== system softMBD/FCS/Controller/position_controller/PID Controller/Anti-windup/Disabled ==
  preInt : Inport  SampleTime=SampleTime
  preSat : Inport  Port=2  SampleTime=SampleTime
  postSat : Inport  Port=3  SampleTime=SampleTime
  P : Inport  Port=4  SampleTime=SampleTime
  Signal Specification1 : SignalSpecification  DisableCoverage=on  OutDataTypeStr=boolean  SampleTime=SampleTime
  Signal Specification2 : SignalSpecification  DisableCoverage=on  OutDataTypeStr=boolean  SampleTime=SampleTime
  Terminator{,1..3} (4 alike) : Terminator
  wires:
  postSat/1 -> Terminator1/1
  Signal Specification2/1 -> Terminator2/1
  P/1 -> Signal Specification2/1
  preSat/1 -> Terminator/1
  preInt/1 -> Signal Specification1/1
  Signal Specification1/1 -> Terminator3/1

== system softMBD/FCS/Controller/position_controller/PID Controller/Anti-windup/Disc. Clamping Ideal ==
  preSat : Inport  SampleTime=SampleTime
  P : Inport  Port=2  SampleTime=SampleTime
  preInt : Inport  Port=3  SampleTime=SampleTime
  postSat : Inport  Port=4  SampleTime=SampleTime
  Upper Limit : Inport  Port=5  SampleTime=SampleTime
  Lower Limit : Inport  Port=6  SampleTime=SampleTime
  AND1 : Logic  DisableCoverage=on  OutDataTypeStr=boolean
  AND2 : Logic  DisableCoverage=on  OutDataTypeStr=boolean
  AND3 : Logic  DisableCoverage=on  OutDataTypeStr=boolean
  Clamping_zero : Constant  DisableCoverage=on  Value=0  OutMin=ClampingZeroOutMin  OutMax=ClampingZeroOutMax  OutDataTypeStr=Inherit: Inherit via back propagation
  Constant1 : Constant  DisableCoverage=on  Value=0  OutDataTypeStr=Inherit: Inherit via back propagation  PreserveConstantTs=on
  Constant4 : Constant  DisableCoverage=on  OutDataTypeStr=int8
  Constant5 : Constant  DisableCoverage=on  Value=-1  OutDataTypeStr=int8
  Constant6 : Constant  DisableCoverage=on  OutDataTypeStr=int8
  Constant7 : Constant  DisableCoverage=on  Value=-1  OutDataTypeStr=int8
  Dead Zone : Subsystem  Variant=on  VariantControlMode=label  LabelModeActiveChoice=Enabled  EmptyChoice=on
  Equal1 : RelationalOperator  DisableCoverage=on  Operator===  OutDataTypeStr=boolean  RndMeth=Floor  InputSameDT=off
  NOT1 : Logic  DisableCoverage=on  Operator=NOT  OutDataTypeStr=boolean
  NOT2 : Logic  DisableCoverage=on  Operator=NOT  OutDataTypeStr=boolean
  OR1 : Logic  DisableCoverage=on  Operator=OR  OutDataTypeStr=boolean
  Relational Operator : RelationalOperator  DisableCoverage=on  Operator=~=  OutDataTypeStr=boolean  RndMeth=Simplest  InputSameDT=off
  Relational Operator1 : RelationalOperator  DisableCoverage=on  Operator=>  OutDataTypeStr=boolean  RndMeth=Simplest  InputSameDT=off
  Switch : Switch  Criteria=u2 > Threshold  SaturateOnIntegerOverflow=off
  Switch2 : Switch  DisableCoverage=on  Criteria=u2 > Threshold  SaturateOnIntegerOverflow=off  InputSameDT=off
  Switch3 : Switch  DisableCoverage=on  Criteria=u2 > Threshold  SaturateOnIntegerOverflow=off  InputSameDT=off
  Terminator1 : Terminator
  fix for DT propagation issue : RelationalOperator  DisableCoverage=on  Operator=>  OutDataTypeStr=boolean  RndMeth=Simplest  InputSameDT=off
  fix for DT propagation issue1 : RelationalOperator  DisableCoverage=on  Operator=>  OutDataTypeStr=boolean  RndMeth=Simplest  InputSameDT=off
  Out1 : Outport  SampleTime=SampleTime
  wires:
  fix for DT propagation issue1/1 -> Switch2/2
  P/1 -> Relational Operator1/1
  Relational Operator/1 -> AND3/1
  Dead Zone/1(DZ out) -> Relational Operator/2, fix for DT propagation issue/1
  fix for DT propagation issue/1 -> Switch3/2
  Clamping_zero/1 -> fix for DT propagation issue/2, fix for DT propagation issue1/2, Relational Operator1/2, Relational Operator/1
  Switch2/1 -> Equal1/2
  Switch3/1 -> Equal1/1
  Constant7/1 -> Switch3/3
  Constant6/1 -> Switch3/1
  Constant4/1 -> Switch2/1
  Constant5/1 -> Switch2/3
  Lower Limit/1 -> Dead Zone/3(Lower Limit)
  Upper Limit/1 -> Dead Zone/2(Upper Limit)
  Switch/1 -> Out1/1
  AND3/1 -> Switch/2
  Constant1/1 -> Switch/1
  OR1/1 -> AND3/2
  AND2/1 -> OR1/2
  AND1/1 -> OR1/1
  NOT2/1 -> AND2/2
  NOT1/1 -> AND2/1
  Relational Operator1/1 -> NOT2/1, AND1/2
  Equal1/1 -> AND1/1, NOT1/1
  preInt/1 -> fix for DT propagation issue1/1, Switch/3
  preSat/1 -> Dead Zone/1(preSat)
  postSat/1 -> Terminator1/1

== system softMBD/FCS/Controller/position_controller/PID Controller/Anti-windup/Disc. Clamping Parallel ==
  preSat : Inport  SampleTime=SampleTime
  preInt : Inport  Port=2  SampleTime=SampleTime
  postSat : Inport  Port=3  SampleTime=SampleTime
  P : Inport  Port=4  SampleTime=SampleTime
  Upper Limit : Inport  Port=5  SampleTime=SampleTime
  Lower Limit : Inport  Port=6  SampleTime=SampleTime
  AND3 : Logic  DisableCoverage=on  OutDataTypeStr=boolean
  Clamping_zero : Constant  DisableCoverage=on  Value=0  OutMin=ClampingZeroOutMin  OutMax=ClampingZeroOutMax  OutDataTypeStr=Inherit: Inherit via back propagation
  Constant : Constant  DisableCoverage=on  OutDataTypeStr=int8
  Constant1 : Constant  DisableCoverage=on  Value=0  OutDataTypeStr=Inherit: Inherit via back propagation  PreserveConstantTs=on
  Constant2 : Constant  DisableCoverage=on  Value=-1  OutDataTypeStr=int8
  Constant3 : Constant  DisableCoverage=on  OutDataTypeStr=int8
  Constant4 : Constant  DisableCoverage=on  Value=-1  OutDataTypeStr=int8
  Dead Zone : Subsystem  Variant=on  VariantControlMode=label  LabelModeActiveChoice=Enabled  EmptyChoice=on
  Equal1 : RelationalOperator  DisableCoverage=on  Operator===  OutDataTypeStr=boolean  RndMeth=Floor  InputSameDT=off
  Relational Operator : RelationalOperator  DisableCoverage=on  Operator=~=  OutDataTypeStr=boolean  RndMeth=Simplest  InputSameDT=off
  Signal Specification2 : SignalSpecification  DisableCoverage=on  OutDataTypeStr=boolean  SampleTime=SampleTime
  Switch : Switch  Criteria=u2 > Threshold  SampleTime=SampleTime  SaturateOnIntegerOverflow=off
  Switch1 : Switch  DisableCoverage=on  Criteria=u2 > Threshold  SaturateOnIntegerOverflow=off  InputSameDT=off
  Switch2 : Switch  DisableCoverage=on  Criteria=u2 > Threshold  SaturateOnIntegerOverflow=off  InputSameDT=off
  Terminator1 : Terminator
  Terminator2 : Terminator
  fix for DT propagation issue : RelationalOperator  DisableCoverage=on  Operator=>  OutDataTypeStr=boolean  RndMeth=Simplest  InputSameDT=off
  fix for DT propagation issue1 : RelationalOperator  DisableCoverage=on  Operator=>  OutDataTypeStr=boolean  RndMeth=Simplest  InputSameDT=off
  Out1 : Outport  SampleTime=SampleTime
  wires:
  fix for DT propagation issue1/1 -> Switch2/2
  fix for DT propagation issue/1 -> Switch1/2
  Clamping_zero/1 -> fix for DT propagation issue/2, fix for DT propagation issue1/2, Relational Operator/1
  Constant1/1 -> Switch/1
  Switch2/1 -> Equal1/2
  Constant3/1 -> Switch2/1
  Constant4/1 -> Switch2/3
  Switch1/1 -> Equal1/1
  preInt/1 -> Switch/3, fix for DT propagation issue1/1
  Constant2/1 -> Switch1/3
  Constant/1 -> Switch1/1
  Relational Operator/1 -> AND3/1
  Lower Limit/1 -> Dead Zone/3(Lower Limit)
  Upper Limit/1 -> Dead Zone/2(Upper Limit)
  preSat/1 -> Dead Zone/1(preSat)
  Dead Zone/1(DZ out) -> Relational Operator/2, fix for DT propagation issue/1
  Equal1/1 -> AND3/2
  AND3/1 -> Switch/2
  Switch/1 -> Out1/1
  Signal Specification2/1 -> Terminator2/1
  postSat/1 -> Terminator1/1
  P/1 -> Signal Specification2/1

== system softMBD/FCS/Controller/position_controller/PID Controller/Anti-windup/Passthrough ==
  preInt : Inport  SampleTime=SampleTime
  preSat : Inport  Port=2  SampleTime=SampleTime
  postSat : Inport  Port=3  SampleTime=SampleTime
  P : Inport  Port=4  SampleTime=SampleTime
  Signal Specification2 : SignalSpecification  DisableCoverage=on  OutDataTypeStr=boolean  SampleTime=SampleTime
  Terminator : Terminator
  Terminator1 : Terminator
  Terminator2 : Terminator
  Out1 : Outport  SampleTime=SampleTime
  wires:
  preInt/1 -> Out1/1
  preSat/1 -> Terminator/1
  postSat/1 -> Terminator1/1
  P/1 -> Signal Specification2/1
  Signal Specification2/1 -> Terminator2/1

== system softMBD/FCS/Controller/position_controller/PID Controller/D Gain/Disabled ==
  D Gain : Inport  SampleTime=SampleTime
  Signal Specification : SignalSpecification  DisableCoverage=on  OutDataTypeStr=boolean  SampleTime=SampleTime
  Terminator : Terminator
  wires:
  D Gain/1 -> Signal Specification/1
  Signal Specification/1 -> Terminator/1

== system softMBD/FCS/Controller/position_controller/PID Controller/D Gain/External Parameters ==
  err : Inport  SampleTime=SampleTime
  D Gain : Inport  Port=2  SampleTime=SampleTime
  DProd Out : Product  OutMin=DOutMin  OutMax=DOutMax  SampleTime=SampleTime
  Out1 : Outport  SampleTime=SampleTime
  wires:
  DProd Out/1 -> Out1/1
  D Gain/1 -> DProd Out/2
  err/1 -> DProd Out/1

== system softMBD/FCS/Controller/position_controller/PID Controller/D Gain/Internal Parameters ==
  err : Inport  SampleTime=SampleTime
  D Gain : Inport  Port=2  SampleTime=SampleTime
  Derivative Gain : Gain  DisableCoverage=on  Gain=D  ParamMin=DParamMin  ParamMax=DParamMax  OutMin=DOutMin  OutMax=DOutMax
  Signal Specification : SignalSpecification  DisableCoverage=on  OutDataTypeStr=boolean  SampleTime=SampleTime
  Terminator : Terminator
  Out1 : Outport  SampleTime=SampleTime
  wires:
  Derivative Gain/1 -> Out1/1
  err/1 -> Derivative Gain/1
  D Gain/1 -> Signal Specification/1
  Signal Specification/1 -> Terminator/1

== system softMBD/FCS/Controller/position_controller/PID Controller/External Derivative/Disabled ==
  ydot : Inport  SampleTime=SampleTime
  err : Inport  Port=2  SampleTime=SampleTime
  Signal Specification : SignalSpecification  DisableCoverage=on  OutDataTypeStr=boolean  SampleTime=SampleTime
  Terminator1 : Terminator
  Out1 : Outport  SampleTime=SampleTime
  wires:
  err/1 -> Terminator1/1
  Signal Specification/1 -> Out1/1
  ydot/1 -> Signal Specification/1

== system softMBD/FCS/Controller/position_controller/PID Controller/External Derivative/Error ==
  err : Inport  SampleTime=SampleTime
  ydot : Inport  Port=2  SampleTime=SampleTime
  Signal Specification : SignalSpecification  DisableCoverage=on  OutDataTypeStr=boolean  SampleTime=SampleTime
  Terminator : Terminator
  Out1 : Outport  SampleTime=SampleTime
  wires:
  Signal Specification/1 -> Terminator/1
  ydot/1 -> Signal Specification/1
  err/1 -> Out1/1
